simulink model "adc"  (R2022b)
settings: Solver=VariableStepAuto  StartTime=0.0  StopTime=1  RelTol=1e-3
libraries: instrumentseriallib x2
settings Model: SimulationMode=accelerator  Creator=ASUS  LastModifiedBy=ASUS

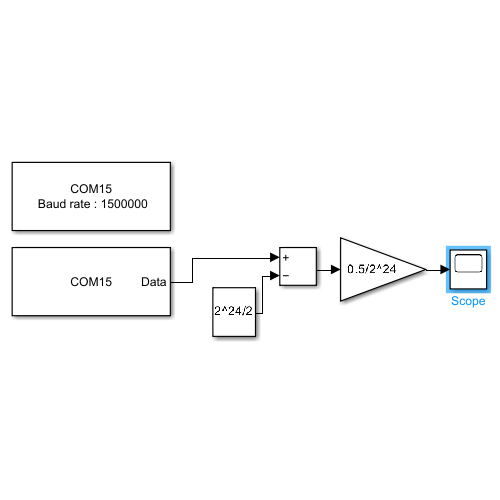
[thumbnail: Simulink's stored preview of the top-level diagram]
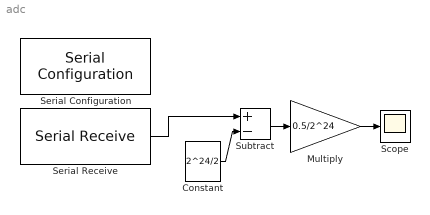
== system adc ==
  Constant : Constant  Value=2^24/2
  Multiply : Gain  Gain=0.5/2^24
  Scope : Scope
  Serial Configuration : instrumentseriallib/Serial Configuration  Priority=-200000  PortSel=COM15  Port=COM15  ComPort=COM15  BaudRate=1500000  DataBits=8  Parity=none  StopBits=1  ByteOrder=little-endian  FlowControl=none  Timeout=1000000  SimulateUsing=Interpreted execution  BlockInModel=on  aMode=1
  Serial Receive : instrumentseriallib/Serial Receive  Priority=1  PortSel=COM15  Port=COM15  ComPort=COM15  DataType=uint32  SaveDataType=uint8  ToggleHeader=off  Header=[]  ToggleTerminator=on  Terminator=Custom terminator  CustomTerminator=[0xA5]  InputFormat=Column major  ToggleDataSize=on  DataSize=[1 2]  EnableBlockingMode=on  ActionDataUnavailable=Output last received value  ActionWhenDataUnavailable=Output last received value  CustomValue=0  SampleTime=1/(16550/2)  SimulateUsing=Interpreted execution  BlockInModel=on  aMode=1
  Subtract : Sum  Inputs=+-
  wires:
  Subtract/1 -> Multiply/1
  Serial Receive/1 -> Subtract/1
  Constant/1 -> Subtract/2
  Multiply/1 -> Scope/1
